simulink model "main_RI_LIEKF_GNSSOutrage"  (R2023a)
settings: Solver=FixedStepAuto  StartTime=0.0  StopTime=220  FixedStep=0.01  RelTol=1e-3
InitFcn:
  | initNavigation0612_AOA;
values from neighbouring files (symbols this model uses):
  CF_enable = 0    [initNavigation.m]
  dt = 0.01    [initNavigation.m]
  dtDelay = -0.03    [initNavigation.m]
  g0 = 9.795    [initNavigation.m]
  gam0_rad = 0/57.3    (= 0)    [initNavigation.m]
  GNSSoutragetime = 90    [initNavigation.m]
  H_sensor_type = 0    [initNavigation.m]
  KF_enable = 1    [initNavigation.m]
  P0 = diag([1*ones(3,1);0.01*ones(3,1);0.1*ones(3,1);0.001*ones(3,1);0.00001*ones(3,1)])    [initNavigation.m]
  P0_RIEKF = diag([1*ones(3,1);0.01*ones(3,1);0.1*ones(3,1);0.001*ones(3,1);0.00001*ones(3,1);      0.01*ones(3,1);[0;2;2]/57.3;[0.1;0.1;0.1]])^2    [initNavigation.m]
  pd0 = 0    [initNavigation.m]
  pe0 = 0    [initNavigation.m]
  phi0_rad = 0/57.3    (= 0)    [initNavigation.m]
  pn0 = 0    [initNavigation.m]
  psi = -178    [initNavigation.m]
  psi0_rad = 0/57.3    (= 0)    [initNavigation.m]
  state_dim = 24    [initNavigation.m]
  Time = 0:0.01:(size(traindata.AttackAngle,1) - 1)*0.01    [NNLiftCoefficientFit.m]
  vd0 = 0    [initNavigation.m]
  ve0 = 0    [initNavigation.m]
  vn0 = 0    [initNavigation.m]
undefined symbols (not defined in the file or in its folder): DiscIntNeverNeededParam, Discrete, INS_CONST, INS_EXPORT, INS_PARAM, magnitude, p, param, pInitialization, sys
libraries: simulink_extras x94, simulink x82, dspstat3 x70, sharedtransform x60, ctrlSharedLib x36, sharedTrackingLibrary x22, matrix_library x15, FMT_Model_Lib x13, deeplib x8, dspsolvers x4, vrlib x4, aerolibconvert2 x1
(part 15 of 28)

== system main_RI_LIEKF_GNSSOutrage/State estimation/distribute CF/distribute CF/AHRS1 ==
  RF_Data : Inport
  Sensor_Data : Inport  Port=2
  Bus_Constructor : Subsystem  TreatAsAtomicUnit=on
  Correct : Subsystem  TreatAsAtomicUnit=on
  Delay : Delay  DelayLength=1
  Update : Subsystem  TreatAsAtomicUnit=on
  Rotation_Data : Outport
  wires:
  Correct/1(att_B_correction) -> Update/1(att_B_correction)
  Bus_Constructor/1(Rotation_Data) -> Delay/1, Rotation_Data/1
  Correct/2(bias_g_B_correction) -> Update/2(bias_g_correction)
  Sensor_Data/1 -> Bus_Constructor/5(Sensor_Data), Update/4(Sensor_Data), Correct/2(Sensor_Data)
  Update/1(att_quat) -> Bus_Constructor/2(att_quat)
  Update/2(DCM_OB) -> Bus_Constructor/3(DCM_OB)
  Update/3(bias_g) -> Bus_Constructor/4(bias_g)
  RF_Data/1 -> Correct/3(RF_Data), Bus_Constructor/1(RF_Data), Update/3(RF_Data)
  Delay/1 -> Correct/1(Rotation_Data)

== system main_RI_LIEKF_GNSSOutrage/State estimation/distribute CF/distribute CF/Bus_Constructor ==
  RF_Data : Inport
  att_quat : Inport  Port=2
  DCM_OB : Inport  Port=3
  bias_g : Inport  Port=4
  gyro_B_correction : Inport  Port=5
  Sensor_Data : Inport  Port=6
  Bus Creator : BusCreator  Inputs=12
  Bus Selector : BusSelector  OutputSignals=IMU_Data.gyro_B_rad/s_LPF,IMU_Data.accl_B_m/s2_LPF
  Bus Selector1 : BusSelector  OutputSignals=att_reset
  Constant : Constant
  Euler_Angle : Subsystem
  Math Function : Math  Operator=transpose  SignedPower=on
  Signal Conversion{,1..4} (5 alike) : SignalConversion  OverrideOpt=off
  Subsystem1 : Subsystem
  Terminator2 : Terminator
  Rotation_Data : Outport
  wires:
  Bus Selector1/1 -> Signal Conversion4/1  "<att_reset>"
  Signal Conversion/1 -> Bus Creator/11  "acc_B_mPs2"
  Euler_Angle/1(phi_rad) -> Bus Creator/2  "phi_rad"
  Euler_Angle/2(theta_rad) -> Bus Creator/3  "theta_rad"
  Euler_Angle/3(psi_rad) -> Subsystem1/1(psi), Bus Creator/4  "psi_rad"
  Sensor_Data/1 -> Bus Selector/1
  Bus Creator/1 -> Rotation_Data/1
  bias_g/1 -> Signal Conversion3/1
  Math Function/1 -> Bus Creator/7  "M_BO"
  DCM_OB/1 -> Math Function/1, Bus Creator/8  "M_OB"
  att_quat/1 -> Euler_Angle/1(att_quat), Bus Creator/6  "att_quat"
  Subsystem1/1(DCMz) -> Bus Creator/5  "M_CO"
  Signal Conversion1/1 -> Bus Creator/12  "standstill"
  Bus Selector/2 -> Signal Conversion/1  "<accl_B_m/s2_LPF>"
  Signal Conversion2/1 -> Bus Creator/10  "gyr_B_radPs"
  Signal Conversion3/1 -> Bus Creator/9  "bias_g"
  RF_Data/1 -> Bus Selector1/1  "att_reset"
  gyro_B_correction/1 -> Signal Conversion2/1
  Signal Conversion4/1 -> Bus Creator/1  "att_reset"
  Constant/1 -> Signal Conversion1/1
  Bus Selector/1 -> Terminator2/1  "<gyro_B_rad/s_LPF>"

== system main_RI_LIEKF_GNSSOutrage/State estimation/distribute CF/distribute CF/Correct ==
  Sensor_Data : Inport
  Rotation_Data : Inport  Port=2
  Attitude_Correction : Subsystem
  Subsystem2 : Subsystem
  att_B_correction : Outport
  bias_g_B_correction : Outport  Port=2
  wires:
  Attitude_Correction/1(att_B_correction) -> att_B_correction/1, Subsystem2/2(att_B_correction)
  Sensor_Data/1 -> Subsystem2/1(Sensor_Data), Attitude_Correction/1(Sensor_Data)
  Subsystem2/1(bias_g_B_correction) -> bias_g_B_correction/1
  Rotation_Data/1 -> Attitude_Correction/2(Rotation_Data)

== system main_RI_LIEKF_GNSSOutrage/State estimation/distribute CF/distribute CF/Translation_estimate ==
  RotationData : Inport
  Sensor_data : Inport  Port=2
  Add : Sum  Inputs=++-
  Bus Creator2 : BusCreator  Inputs=6
  Bus Selector : BusSelector  OutputSignals=TOF_Data.H_TOF_TD,GPS_Data.pos_D_gps,QGC_sensor_reinit,GPS_Data.fixtype_gps
  Bus Selector1 : BusSelector  OutputSignals=M_OB
  Compare To Constant : simulink/Logic and Bit Operations/Compare To Constant  relop=>=  const=1  OutDataTypeStr=boolean
  Constant2 : Constant  Value=g0  OutDataTypeStr=single
  Demux : Demux  Outputs=2
  Demux1 : Demux  Outputs=2
  Demux2 : Demux  Outputs=3
  Detect Increase : simulink/Logic and Bit Operations/Detect Increase  vinit=0.0  OutDataTypeStr=boolean
  Gain : Gain  Gain=-1
  KalmanFilter_altitude : ctrlSharedLib/Kalman Filter  TimeDomain=Discrete-Time  UseCurrentEstimator=on  ModelSource=Individual A, B, C, D matrices  ModelSourceVariable=sys  A=[1 0.01 0; 0 1 -0.01;0 0 1-1/50;]  B=[0;0.01;0]  C=[1 0 0]  D=[0]  NumberOfStates=2  NumberOfInputs=2  NumberOfOutputs=2  InitialEstimateSource=Dialog  X0=[0 0 0]  P0=10  UseK=off  UseGH=on  NumberOfProcessNoiseInputs=2  G=diag([0;1;1])  TimeInvariantG=on  H=0  TimeInvariantH=on  Q=diag([0;5e-3;5e-4])  TimeInvariantQ=on  R=10  TimeInvariantR=on  N=0  TimeInvariantN=on  AddInputPort=on  AddEnablePort=on  ExternalReset=Rising  OutputEstimatedY=off  OutputP=off  Ts=-1
  Memory : Memory
  Rxy_Horizontal_estimation : Subsystem
  Scope : Scope  NumInputPorts=2
  Sensor_data1 : InportShadow  Port=2
  V_Horizontal_estimation : Subsystem
  Zero-Order Hold{,1..3} (4 alike) : ZeroOrderHold  SampleTime=0.01
  translate to N : Subsystem
  TranslationData : Outport
  wires:
  RotationData/1 -> Bus Selector1/1, translate to N/1(RotationData)
  Bus Creator2/1 -> TranslationData/1
  Demux1/2 -> Bus Creator2/5  "pe_m"
  Demux1/1 -> Bus Creator2/4  "pn_m"
  Demux/2 -> Bus Creator2/2  "ve_m/s"
  Demux/1 -> Bus Creator2/1  "vn_m/s"
  translate to N/2(accel_Vertical_predict) -> [accel_Vertical_predict]
  V_Horizontal_estimation/3(GPS_v_enable) -> Rxy_Horizontal_estimation/2(Enable)
  V_Horizontal_estimation/2(V_n&e) -> Rxy_Horizontal_estimation/1(Vn)
  V_Horizontal_estimation/1(vxy_estimout) -> Demux/1  "v_ne_"
  translate to N/1(accel_Horizontal_predict) -> V_Horizontal_estimation/1(An)
  Rxy_Horizontal_estimation/1(R_n&e) -> Demux1/1
  Sensor_data/1 -> translate to N/2(Sensor_data), V_Horizontal_estimation/2(Sensor_data2), Rxy_Horizontal_estimation/3(Sensor_data2)
  Sensor_data1/1 -> Bus Selector/1
  KalmanFilter_altitude/1 -> Demux2/1
  Demux2/1 -> Gain/1
  Zero-Order Hold/1 -> KalmanFilter_altitude/1
  Zero-Order Hold1/1 -> KalmanFilter_altitude/2
  Demux2/2 -> Bus Creator2/3  "vd_m/s"
  Gain/1 -> Bus Creator2/6  "H_m"
  [accel_Vertical_predict] -> Scope/1, Add/1
  Add/1 -> Zero-Order Hold/1
  Demux2/3 -> Memory/1
  Memory/1 -> Add/3, Scope/2
  Constant2/1 -> Add/2
  Bus Selector/3 -> Detect Increase/1  "<QGC_sensor_reinit>"
  Detect Increase/1 -> Zero-Order Hold3/1
  Bus Selector/4 -> Zero-Order Hold2/1  "<fixtype_gps>"
  Compare To Constant/1 -> KalmanFilter_altitude/3
  Zero-Order Hold2/1 -> Compare To Constant/1
  Bus Selector/2 -> Zero-Order Hold1/1  "<pos_D_gps>"
  Zero-Order Hold3/1 -> KalmanFilter_altitude/4
  Bus Selector1/1 -> Rxy_Horizontal_estimation/4(Cbn)  "<M_OB>"

== system main_RI_LIEKF_GNSSOutrage/State estimation/distribute CF/distribute CF/Update ==
  note: 比例环节
  att_B_correction : Inport
  bias_g_correction : Inport  Port=2
  RF_Data : Inport  Port=3
  Sensor_Data : Inport  Port=4
  Attitude_Update : Subsystem
  Bus Selector : BusSelector  OutputSignals=IMU_Data.gyro_B_rad/s_LPF
  Bus Selector1 : BusSelector  OutputSignals=att_reset,quat_0
  Gain : Gain
  Gyro_Bias_Update : Subsystem
  Saturation : Saturate  UpperLimit=0.1  LowerLimit=-0.1
  Scope : Scope
  Scope1 : Scope
  Sum2 : Sum  Inputs=|++
  att_quat : Outport
  DCM_OB : Outport  Port=2
  bias_g : Outport  Port=3
  gyro_B_correction : Outport  Port=4
  wires:
  Sensor_Data/1 -> Bus Selector/1
  Sum2/1 -> Attitude_Update/3(att_B_correction)
  Bus Selector/1 -> Gyro_Bias_Update/2(gyr_B_radPs)  "<gyro_B_rad/s_LPF>"
  bias_g_correction/1 -> Gyro_Bias_Update/1(bias_g_correction)
  Attitude_Update/1(att_quat) -> att_quat/1
  Attitude_Update/2(DCM_OB) -> DCM_OB/1
  Gyro_Bias_Update/2(bias_g) -> Scope/1, bias_g/1
  RF_Data/1 -> Bus Selector1/1  "att_reset"
  Bus Selector1/1 -> Attitude_Update/1(att_reset)  "<att_reset>"
  Bus Selector1/2 -> Attitude_Update/2(quat_0)  "<quat_0>"
  Gyro_Bias_Update/1(gyr_B_correction) -> gyro_B_correction/1, Sum2/2
  att_B_correction/1 -> Gain/1
  Gain/1 -> Saturation/1, Scope1/1
  Saturation/1 -> Sum2/1

== system main_RI_LIEKF_GNSSOutrage/State estimation/distribute CF/distribute CF/初始化 ==
  Sensor_Data : Inport
  Attitude_Reset : Subsystem
  Bus Creator : BusCreator  Inputs=2
  Scope : Scope
  Scope1 : Scope
  Subsystem : Subsystem
  RF_data : Outport
  wires:
  Attitude_Reset/1(att_reset) -> Subsystem/Enable, Bus Creator/1, Scope/1  "att_reset"
  Bus Creator/1 -> RF_data/1
  Subsystem/1(quat_0) -> Scope1/1, Bus Creator/2  "quat_0"
  Sensor_Data/1 -> Subsystem/1(sensor_data), Attitude_Reset/1(Sensor_Data)

== system main_RI_LIEKF_GNSSOutrage/Sensor_Data_Process/Magn_Data_Process1/Mag_Data_Process/Mag_Quality_Estimate/Mag_Quality ==
  nominal_inc_deg : Inport
  mag_normalized_O : Inport  Port=2
  Inclination_Quality_Estimate : Subsystem
  Intensity_Quality_Estimate : Subsystem
  MinMax : MinMax  Inputs=2
  低通滤波 : Subsystem  mask{fc=5, zeta=0.707}
      mask prompts: fc "Cut-off frequence"; zeta "Damping factor"
      mask DialogControl ParameterGroupVar Prompt: 参数
  mag_quality : Outport  PortDimensions=1  VectorParamsAs1DForOutWhenUnconnected=off
  wires:
  Intensity_Quality_Estimate/1(intensity_quality) -> MinMax/2  "mag_int_quality"
  nominal_inc_deg/1 -> Inclination_Quality_Estimate/1(nominal_inc_deg)
  Inclination_Quality_Estimate/1(inclination_quality) -> MinMax/1  "mag_inc_quality"
  mag_normalized_O/1 -> Inclination_Quality_Estimate/2(mag_normalized_O), Intensity_Quality_Estimate/1(mag_normalized_O)
  MinMax/1 -> 低通滤波/1(u)
  低通滤波/1(y) -> mag_quality/1

== system main_RI_LIEKF_GNSSOutrage/Sensor_Data_Process/Magn_Data_Process1/Mag_Data_Process/WMM_Compensation/Normlize ==
  In1 : Inport
  Constant : Constant  OutDataTypeStr=Inherit: Inherit via back propagation
  Data Type Duplicate : DataTypeDuplicate
  Demux : Demux  Outputs=[-1 1]
  Divide : Product  Inputs=*/
  Ground : Ground
  Math Function : Math  Operator=square  SignedPower=on  OutDataTypeStr=Inherit: Inherit via internal rule
  Math Function1 : Math  Operator=sqrt  SignedPower=on
  Mux : Mux  Inputs=2
  Mux1 : Mux  Inputs=2
  Product : Product  RndMeth=Zero  OutDataTypeStr=Inherit: Same as first input
  Sum of Elements : Sum  Inputs=+
  Switch : Switch  Criteria=u2 > Threshold  SaturateOnIntegerOverflow=off  InputSameDT=off
  Out1 : Outport  PortDimensions=3
  wires:
  Mux/1 -> Switch/1
  Ground/1 -> Product/2
  In1/1 -> Mux/1, Math Function/1, Product/1, Data Type Duplicate/2
  Sum of Elements/1 -> Math Function1/1
  Product/1 -> Mux1/1
  Math Function1/1 -> Switch/2, Mux/2
  Demux/2 -> Divide/2
  Switch/1 -> Demux/1
  Mux1/1 -> Switch/3
  Math Function/1 -> Sum of Elements/1
  Constant/1 -> Mux1/2, Data Type Duplicate/1
  Demux/1 -> Divide/1
  Divide/1 -> Out1/1

== system main_RI_LIEKF_GNSSOutrage/Sensor_Data_Process/Magn_Data_Process1/Mag_Data_Process/WMM_Compensation/psi2DCMz ==
  In1 : Inport
  Constant : Constant  OutDataTypeStr=Inherit: Inherit via back propagation
  Constant{1..4} (4 alike) : Constant  Value=0  OutDataTypeStr=Inherit: Inherit via back propagation
  Gain1 : Gain  Gain=-1
  Trigonometric Function : Trigonometry
  Trigonometric Function1 : Trigonometry  Operator=cos
  Trigonometric Function2 : Trigonometry
  Trigonometric Function3 : Trigonometry  Operator=cos
  Vector Concatenate : Concatenate  NumInputs=3  Mode=Multidimensional array  ConcatenateDimension=2
  Vector Concatenate1 : Concatenate  NumInputs=3  Mode=Multidimensional array
  Vector Concatenate2 : Concatenate  NumInputs=3  Mode=Multidimensional array
  Vector Concatenate3 : Concatenate  NumInputs=3  Mode=Multidimensional array
  Out1 : Outport
  wires:
  Constant1/1 -> Vector Concatenate3/2
  Constant/1 -> Vector Concatenate3/3
  Vector Concatenate/1 -> Out1/1
  Trigonometric Function2/1 -> Gain1/1
  Constant2/1 -> Vector Concatenate3/1
  In1/1 -> Trigonometric Function3/1, Trigonometric Function2/1, Trigonometric Function/1, Trigonometric Function1/1
  Trigonometric Function/1 -> Vector Concatenate1/2
  Vector Concatenate2/1 -> Vector Concatenate/2
  Vector Concatenate1/1 -> Vector Concatenate/1
  Vector Concatenate3/1 -> Vector Concatenate/3
  Gain1/1 -> Vector Concatenate2/1
  Constant3/1 -> Vector Concatenate1/3
  Trigonometric Function1/1 -> Vector Concatenate1/1
  Constant4/1 -> Vector Concatenate2/3
  Trigonometric Function3/1 -> Vector Concatenate2/2

== system main_RI_LIEKF_GNSSOutrage/Sensor_Data_Process/Magn_Data_Process1/Mag_Data_Process/WMM_Compensation/safe_divide ==
  u1 : Inport
  u2 : Inport  Port=2
  Constant1 : Constant  VectorParams1D=off  OutDataTypeStr=single
  Divide1 : Product  Inputs=*/
  MinMax : MinMax  Function=max  Inputs=2
  y : Outport  VectorParamsAs1DForOutWhenUnconnected=off
  wires:
  MinMax/1 -> Divide1/2
  Constant1/1 -> MinMax/1
  Divide1/1 -> y/1
  u2/1 -> MinMax/2
  u1/1 -> Divide1/1

== system main_RI_LIEKF_GNSSOutrage/State estimation/0609bk/Error State Kalman Filter/Extended Kalman Filter1/Correct1 ==
  yMeas : Inport  SampleTime=SampleTime
  R : Inport  Port=2  SampleTime=SampleTime
  uMeas : Inport  Port=3  SampleTime=SampleTime
  uBlockOrdering : Inport  Port=4  SampleTime=SampleTime
  Enable : EnablePort
  Correct : MATLAB Function  TreatAsAtomicUnit=on
  Data Store ReadP : DataStoreRead  DataStoreName=P  IndexOptions=Index vector (dialog)  Indices=1  OutputSizes=1
  Data Store ReadX : DataStoreRead  DataStoreName=x  IndexOptions=Index vector (dialog)  Indices=1  OutputSizes=1
  Data Store WriteP : DataStoreWrite  DataStoreName=P  IndexOptions=Index vector (dialog)  Indices=1  OutputSizes=1
  Data Store WriteX : DataStoreWrite  DataStoreName=x  IndexOptions=Index vector (dialog)  Indices=1  OutputSizes=1
  IGG_check : Subsystem  Commented=on
  R1 : InportShadow  Port=2  SampleTime=SampleTime
  RegisterSimulinkFcn : S-Function  FunctionName=ekfukfRegisterSimulinkFcn  Parameters=int32(3), 1, pM.HasAdditiveNoise, SampleTime, DataType, SLFcnsToRegister  SFunctionDeploymentMode=off  EnableBusSupport=off
  Scope1 : Scope
  yMeas1 : InportShadow  SampleTime=SampleTime
  yBlockOrdering : Outport  VectorParamsAs1DForOutWhenUnconnected=off
  wires:
  uMeas/1 -> Correct/5(uMeas)
  uBlockOrdering/1 -> Correct/6("blockOrdering ")
  Correct/3(blockOrdering) -> yBlockOrdering/1
  Correct/1(xNew) -> Data Store WriteX/1
  R/1 -> RegisterSimulinkFcn/3, Correct/4(R)
  yMeas/1 -> RegisterSimulinkFcn/2, Correct/3(yMeas)
  Correct/2(P) -> Data Store WriteP/1
  Data Store ReadP/1 -> IGG_check/1(Pk/k_1), Correct/2("P ")
  Data Store ReadX/1 -> IGG_check/3(X), Correct/1(x), RegisterSimulinkFcn/1
  yMeas1/1 -> IGG_check/2(yMeas)
  R1/1 -> IGG_check/4(R)
  IGG_check/2(w) -> Scope1/1

== system main_RI_LIEKF_GNSSOutrage/State estimation/0609bk/Error State Kalman Filter/Extended Kalman Filter1/Output ==
  uBlockOrdering : Inport
  Data Store Read : DataStoreRead  DataStoreName=x  IndexOptions=Index vector (dialog)  Indices=1  OutputSizes=1
  Data Store Read1 : DataStoreRead  DataStoreName=P  IndexOptions=Index vector (dialog)  Indices=1  OutputSizes=1
  MATLAB Function : MATLAB Function  TreatAsAtomicUnit=on
  x : Outport  VectorParamsAs1DForOutWhenUnconnected=off
  P : Outport  Port=2  VectorParamsAs1DForOutWhenUnconnected=off
  yBlockOrdering : Outport  Port=3  VectorParamsAs1DForOutWhenUnconnected=off
  wires:
  MATLAB Function/1(P) -> P/1
  uBlockOrdering/1 -> yBlockOrdering/1
  Data Store Read1/1 -> MATLAB Function/1(S)
  Data Store Read/1 -> x/1

== system main_RI_LIEKF_GNSSOutrage/State estimation/0609bk/Error State Kalman Filter/Extended Kalman Filter1/Predict ==
  Q : Inport  SampleTime=SampleTime
  uState : Inport  Port=2  SampleTime=SampleTime
  uBlockOrdering : Inport  Port=3  SampleTime=SampleTime
  Data Store Read1 : DataStoreRead  Commented=on  DataStoreName=feedback_flag_18dim  IndexOptions=Index vector (dialog)  Indices=1  OutputSizes=1
  Data Store Write : DataStoreWrite  DataStoreName=P  IndexOptions=Index vector (dialog)  Indices=1  OutputSizes=1
  Data Store Write1 : DataStoreWrite  DataStoreName=x  IndexOptions=Index vector (dialog)  Indices=1  OutputSizes=1
  Data Store WriteX : DataStoreWrite  DataStoreName=x  IndexOptions=Index vector (dialog)  Indices=1  OutputSizes=1
  Data Store ReadP : DataStoreRead  DataStoreName=P  IndexOptions=Index vector (dialog)  Indices=1  OutputSizes=1
  Data Store ReadX : DataStoreRead  DataStoreName=x  IndexOptions=Index vector (dialog)  Indices=1  OutputSizes=1
  If : If  Commented=on  IfExpression=u1 == 1  ShowElse=off
  If Action Subsystem : Subsystem  Commented=on  TreatAsAtomicUnit=on
  Predict : MATLAB Function  TreatAsAtomicUnit=on
  RegisterSimulinkFcn : S-Function  FunctionName=ekfukfRegisterSimulinkFcn  Parameters=int32(2), 0, pS.HasAdditiveNoise, SampleTime, DataType, SLFcnsToRegister  SFunctionDeploymentMode=off  EnableBusSupport=off
  Zero : Constant  Value=zeros(15,1)  OutDataTypeStr=Inherit: Inherit via back propagation
  wires:
  Zero/1 -> Data Store Write1/1
  If/1 -> If Action Subsystem/Action
  Data Store Read1/1 -> If/1
  uState/1 -> Predict/4(uState)
  uBlockOrdering/1 -> Predict/5(unused)
  Data Store ReadX/1 -> RegisterSimulinkFcn/1, Predict/1(x)
  Predict/1(xNew) -> Data Store WriteX/1
  Q/1 -> RegisterSimulinkFcn/2, Predict/3(Q)
  Predict/2(P) -> Data Store Write/1
  Data Store ReadP/1 -> Predict/2("P ")

== system main_RI_LIEKF_GNSSOutrage/State estimation/0609bk/Error State Kalman Filter/Simulink Function - State Transition/Cal Phi ==
  Rbn : Inport
  vn : Inport  Port=2
  pn : Inport  Port=3
  Constant : Constant  Value=dt
  MATLAB Function1 : MATLAB Function  TreatAsAtomicUnit=on
  Reshape : Reshape  OutputDimensionality=Column vector (2-D)
  Reshape1 : Reshape  OutputDimensionality=Column vector (2-D)
  Phi : Outport
  wires:
  Reshape1/1 -> MATLAB Function1/2(pn)
  Reshape/1 -> MATLAB Function1/1(vn)
  pn/1 -> Reshape1/1
  vn/1 -> Reshape/1
  Rbn/1 -> MATLAB Function1/3(Rbn)
  MATLAB Function1/1(Phi) -> Phi/1
  Constant/1 -> MATLAB Function1/4(dt)

== system main_RI_LIEKF_GNSSOutrage/State estimation/0609bk/INS propogation/Init_PVQ/Horizontal_attitude ==
  note: fai
  note: gamma
  accl_mean_B_m/s_LPF : Inport  PortDimensions=3
  Magn_mean_B_guess_LPF : Inport  Port=2
  Enable : EnablePort
  Add : Sum  Inputs=+-
  Asin : Trigonometry  Operator=asin
  Atan2 : Trigonometry  Operator=atan2
  Data Type Conversion : DataTypeConversion  SaturateOnIntegerOverflow=off  RndMeth=Floor
  Deal with zero : Subsystem
  Degrees to Radians : simulink_extras/Transformations/Degrees to Radians
  Degrees to Radians1 : simulink_extras/Transformations/Degrees to Radians
  Demux : Demux  Outputs=3
  Divide : Product  Inputs=*/  OutDataTypeStr=single
  Gain1 : Gain  Gain=-1
  Gain2 : Gain  Gain=-1
  Magnetic declination : Constant  Value=param.fusion.magDeclDeg  OutDataTypeStr=single
  Magnetic declination1 : Constant  Value=param.control.MagnheadingCorrection  OutDataTypeStr=uint8
  Math Function : Math  Operator=magnitude^2  SignedPower=on
  Mux : Mux  Inputs=3
  Mux1 : Mux  Inputs=3
  Mux3 : Mux  Inputs=3
  Product : Product  Multiplication=Matrix(*)
  Quaternions to Direction Cosine Matrix : sharedtransform/Quaternions to  Direction Cosine Matrix  aMode=aMode
  Rotation Angles to Quaternions : sharedtransform/Rotation Angles to Quaternions  rotationOrder=ZYX  aMode=aMode
  Rotation Angles to Quaternions1 : sharedtransform/Rotation Angles to Quaternions  rotationOrder=ZYX  aMode=aMode
  Scope : Scope
  Scope1 : Scope
  Selector : Selector  InputPortWidth=3  IndexOptions=Index vector (dialog)  Indices=[2]  OutputSizes=1
  Selector1 : Selector  InputPortWidth=3  IndexOptions=Index vector (dialog)  Indices=[1]  OutputSizes=1
  Sqrt : Sqrt
  Sum of Elements : Sum  Inputs=+
  Switch : Switch  Threshold=0.5  SaturateOnIntegerOverflow=off  InputSameDT=off
  Terminator : Terminator
  Transpose : Math  Operator=transpose  SignedPower=on
  Trigonometric Function1 : Trigonometry  Operator=atan2
  psi_zero : Constant  Value=psi  OutDataTypeStr=single
  quat_0 : Outport  PortDimensions=4
  wires:
  Rotation Angles to Quaternions1/1 -> Switch/1
  accl_mean_B_m/s_LPF/1 -> Demux/1
  Sqrt/1 -> Deal with zero/1(In1)
  Deal with zero/1(Out1) -> Divide/2
  Trigonometric Function1/1 -> Gain2/1
  Demux/1 -> Divide/1, Mux/2
  Demux/2 -> Mux/1, Trigonometric Function1/1
  Demux/3 -> Gain1/1
  Sum of Elements/1 -> Sqrt/1
  Divide/1 -> Asin/1
  Mux/1 -> Math Function/1
  Math Function/1 -> Sum of Elements/1
  Mux1/1 -> Rotation Angles to Quaternions/1
  psi_zero/1 -> Degrees to Radians1/1
  Asin/1 -> Mux3/2, Mux1/2
  Gain2/1 -> Mux3/3, Mux1/3
  Rotation Angles to Quaternions/1 -> Switch/3, Quaternions to Direction Cosine Matrix/1  "q0_no_yaw"
  Quaternions to Direction Cosine Matrix/1 -> Transpose/1
  Magn_mean_B_guess_LPF/1 -> Product/2
  Product/1 -> Selector/1, Selector1/1  "magNED"
  Selector1/1 -> Atan2/2  "magN"
  Selector/1 -> Atan2/1  "magE"
  Atan2/1 -> Add/2
  Magnetic declination/1 -> Degrees to Radians/1
  Add/1 -> Mux3/1  "psi_calbymag"
  Mux3/1 -> Rotation Angles to Quaternions1/1
  Transpose/1 -> Product/1
  Gain1/1 -> Trigonometric Function1/2, Mux/3
  Degrees to Radians1/1 -> Mux1/1
  Degrees to Radians/1 -> Terminator/1
  Magnetic declination1/1 -> Data Type Conversion/1, Switch/2
  Switch/1 -> Scope1/1, quat_0/1
  Data Type Conversion/1 -> Scope/1

== system main_RI_LIEKF_GNSSOutrage/State estimation/0609bk/INS propogation/Init_PVQ/Subsystem ==
  data : Inport
  Buffer : Buffer  N=50  V=49  OutputFrames=off
  Buffer1 : Buffer  N=50  V=49  OutputFrames=off
  Buffer2 : Buffer  N=50  V=49  ic=-g0  OutputFrames=off
  Demux : Demux  Outputs=3
  Mean4 : dspstat3/Mean  run=off  reset_popup=None  directionMode=Entire input  dimension=3  roiEnable=off  roiType=Rectangles  roiPortion=Entire ROI  roiOutput=Individual statistics for each ROI  roiFlag=off  roundingMode=Floor  overflowMode=off  outputDataTypeStr=Inherit: Same as accumulator  outputMin=[]  outputMax=[]  outputLastDataTypeStr=Inherit: Same as accumulator
  Mean5 : dspstat3/Mean  run=off  reset_popup=None  directionMode=Entire input  dimension=3  roiEnable=off  roiType=Rectangles  roiPortion=Entire ROI  roiOutput=Individual statistics for each ROI  roiFlag=off  roundingMode=Floor  overflowMode=off  outputDataTypeStr=Inherit: Same as accumulator  outputMin=[]  outputMax=[]  outputLastDataTypeStr=Inherit: Same as accumulator
  Mean6 : dspstat3/Mean  run=off  reset_popup=None  directionMode=Entire input  dimension=3  roiEnable=off  roiType=Rectangles  roiPortion=Entire ROI  roiOutput=Individual statistics for each ROI  roiFlag=off  roundingMode=Floor  overflowMode=off  outputDataTypeStr=Inherit: Same as accumulator  outputMin=[]  outputMax=[]  outputLastDataTypeStr=Inherit: Same as accumulator
  Scope : Scope  NumInputPorts=2
  Vector Concatenate : Concatenate  NumInputs=3
  mean_data : Outport
  wires:
  Mean6/1 -> Vector Concatenate/3
  Demux/2 -> Buffer1/1
  Buffer/1 -> Mean4/1  "fbx_buff"
  Mean5/1 -> Vector Concatenate/2
  Buffer2/1 -> Mean6/1  "fbz_buff"
  Demux/1 -> Buffer/1
  Buffer1/1 -> Mean5/1  "fby_buff"
  Demux/3 -> Buffer2/1
  Mean4/1 -> Vector Concatenate/1
  Vector Concatenate/1 -> Scope/2, mean_data/1
  data/1 -> Scope/1, Demux/1

== system main_RI_LIEKF_GNSSOutrage/State estimation/0609bk/INS propogation/Init_PVQ/Subsystem1 ==
  data : Inport
  Buffer : Buffer  N=50  V=49  OutputFrames=off
  Buffer1 : Buffer  N=50  V=49  OutputFrames=off
  Buffer2 : Buffer  N=50  V=49  OutputFrames=off
  Demux : Demux  Outputs=3
  Mean4 : dspstat3/Mean  run=off  reset_popup=None  directionMode=Entire input  dimension=3  roiEnable=off  roiType=Rectangles  roiPortion=Entire ROI  roiOutput=Individual statistics for each ROI  roiFlag=off  roundingMode=Floor  overflowMode=off  outputDataTypeStr=Inherit: Same as accumulator  outputMin=[]  outputMax=[]  outputLastDataTypeStr=Inherit: Same as accumulator
  Mean5 : dspstat3/Mean  run=off  reset_popup=None  directionMode=Entire input  dimension=3  roiEnable=off  roiType=Rectangles  roiPortion=Entire ROI  roiOutput=Individual statistics for each ROI  roiFlag=off  roundingMode=Floor  overflowMode=off  outputDataTypeStr=Inherit: Same as accumulator  outputMin=[]  outputMax=[]  outputLastDataTypeStr=Inherit: Same as accumulator
  Mean6 : dspstat3/Mean  run=off  reset_popup=None  directionMode=Entire input  dimension=3  roiEnable=off  roiType=Rectangles  roiPortion=Entire ROI  roiOutput=Individual statistics for each ROI  roiFlag=off  roundingMode=Floor  overflowMode=off  outputDataTypeStr=Inherit: Same as accumulator  outputMin=[]  outputMax=[]  outputLastDataTypeStr=Inherit: Same as accumulator
  Vector Concatenate : Concatenate  NumInputs=3
  mean_data : Outport
  wires:
  data/1 -> Demux/1
  Vector Concatenate/1 -> mean_data/1
  Mean4/1 -> Vector Concatenate/1
  Demux/3 -> Buffer2/1
  Buffer1/1 -> Mean5/1  "fby_buff"
  Demux/1 -> Buffer/1
  Buffer2/1 -> Mean6/1  "fbz_buff"
  Mean5/1 -> Vector Concatenate/2
  Buffer/1 -> Mean4/1  "fbx_buff"
  Demux/2 -> Buffer1/1
  Mean6/1 -> Vector Concatenate/3

== system main_RI_LIEKF_GNSSOutrage/State estimation/0609bk/INS propogation/vel_pos_update/Kinematic Equation ==
  Cbn : Inport
  Ab : Inport  Port=2
  Add : Sum  Inputs=+-
  Constant : Constant  Value=[0 0 -g0]  OutDataTypeStr=single
  Product : Product  Multiplication=Matrix(*)  RndMeth=Zero
  Scope : Scope
  Scope1 : Scope  NumInputPorts=2
  An : Outport
  wires:
  Cbn/1 -> Product/1
  Add/1 -> An/1, Scope1/2
  Ab/1 -> Product/2, Scope1/1
  Product/1 -> Scope/1, Add/1
  Constant/1 -> Add/2

== system main_RI_LIEKF_GNSSOutrage/State estimation/0609bk/INS propogation/vel_pos_update/pos update ==
  vel_k : Inport
  pn : Inport  Port=2
  QGC_init : Inport  Port=3
  p0 : Inport  Port=4
  Add1 : Sum
  Delay1 : Delay  DelayLength=1  InitialConditionSource=Input port  ExternalReset=Rising
      settings: InputPortMap=u0,r5,p4
  Gain1 : Gain  Gain=dt
  Reshape1 : Reshape  OutputDimensionality=Column vector (2-D)
  p_k : Outport
  wires:
  p0/1 -> Reshape1/1
  QGC_init/1 -> Delay1/2
  Reshape1/1 -> Delay1/3
  Delay1/1 -> Add1/2
  Gain1/1 -> Add1/1
  vel_k/1 -> Gain1/1
  Add1/1 -> p_k/1
  pn/1 -> Delay1/1

== system main_RI_LIEKF_GNSSOutrage/State estimation/0609bk/INS propogation/vel_pos_update/vel update ==
  QGC_init : Inport
  An : Inport  Port=2
  vn : Inport  Port=3
  v0 : Inport  Port=4
  Add : Sum
  Delay : Delay  DelayLength=1  InitialConditionSource=Input port  ExternalReset=Rising
      settings: InputPortMap=u0,r5,p4
  Gain : Gain  Gain=dt
  Reshape : Reshape  OutputDimensionality=Column vector (2-D)
  vel_k : Outport
  wires:
  QGC_init/1 -> Delay/2
  Reshape/1 -> Delay/3
  An/1 -> Gain/1
  v0/1 -> Reshape/1
  Gain/1 -> Add/1
  Delay/1 -> Add/2
  Add/1 -> vel_k/1
  vn/1 -> Delay/1

== system main_RI_LIEKF_GNSSOutrage/State estimation/15dim KF1/Error State Kalman Filter/GNSS//INS Kalman Filter1/CalculatePL ==
  A[k] : Inport  SampleTime=pInitialization.Ts
  C[k] : Inport  Port=2  SampleTime=pInitialization.Ts
  Qbar[k] : Inport  Port=3  SampleTime=pInitialization.Ts
  Rbar[k] : Inport  Port=4  SampleTime=pInitialization.Ts
  Nbar[k] : Inport  Port=5  SampleTime=pInitialization.Ts
  Enable[k] : Inport  Port=6  SampleTime=pInitialization.Ts
  P[k] : Inport  Port=7  SampleTime=pInitialization.Ts
  Discrete-Time KF - Calculate PLMZ : MATLAB Function  TreatAsAtomicUnit=on
  M[k] : Outport  SampleTime=pInitialization.Ts  VectorParamsAs1DForOutWhenUnconnected=off
  L[k] : Outport  Port=2  SampleTime=pInitialization.Ts  VectorParamsAs1DForOutWhenUnconnected=off
  Z[k] : Outport  Port=3  SampleTime=pInitialization.Ts  VectorParamsAs1DForOutWhenUnconnected=off
  P[k+1] : Outport  Port=4  SampleTime=pInitialization.Ts  VectorParamsAs1DForOutWhenUnconnected=off
  wires:
  A[k]/1 -> Discrete-Time KF - Calculate PLMZ/1(A)
  C[k]/1 -> Discrete-Time KF - Calculate PLMZ/2(C)
  Qbar[k]/1 -> Discrete-Time KF - Calculate PLMZ/3(Q)
  P[k]/1 -> Discrete-Time KF - Calculate PLMZ/6(P)
  Rbar[k]/1 -> Discrete-Time KF - Calculate PLMZ/4(R)
  Nbar[k]/1 -> Discrete-Time KF - Calculate PLMZ/5(N)
  Discrete-Time KF - Calculate PLMZ/1(L) -> L[k]/1
  Discrete-Time KF - Calculate PLMZ/4(PNew) -> P[k+1]/1
  Enable[k]/1 -> Discrete-Time KF - Calculate PLMZ/7(isEnabled)
  Discrete-Time KF - Calculate PLMZ/2(M) -> M[k]/1
  Discrete-Time KF - Calculate PLMZ/3(Z) -> Z[k]/1

== system main_RI_LIEKF_GNSSOutrage/State estimation/15dim KF1/Error State Kalman Filter/GNSS//INS Kalman Filter1/CovarianceOutputConfigurator ==
  Z : Inport
  P : Inport  Port=2
  TerminatorP : Terminator
  TerminatorZ : Terminator
  decideOutput : Subsystem  mask(outputZorP){}
  Covariance : Outport  VectorParamsAs1DForOutWhenUnconnected=off
  wires:
  decideOutput/1(P) -> Covariance/1
  P/1 -> TerminatorP/1, decideOutput/1(Z)
  Z/1 -> TerminatorZ/1

== system main_RI_LIEKF_GNSSOutrage/State estimation/15dim KF1/Error State Kalman Filter/GNSS//INS Kalman Filter1/If Action Subsystem1 ==
  x[k+1|k] : Inport
  Action Port : ActionPort
  Constant : Constant  Value=0
  Data Store Write : DataStoreWrite  DataStoreName=feedback_flag  IndexOptions=Index vector (dialog)  Indices=1  OutputSizes=1
  Gain : Gain  Gain=0
  Out1 : Outport
  wires:
  Constant/1 -> Data Store Write/1
  Gain/1 -> Out1/1
  x[k+1|k]/1 -> Gain/1

== system main_RI_LIEKF_GNSSOutrage/State estimation/15dim KF1/Error State Kalman Filter/GNSS//INS Kalman Filter1/If Action Subsystem2 ==
  x[k+1|k] : Inport
  Action Port : ActionPort
  Out1 : Outport
  wires:
  x[k+1|k]/1 -> Out1/1

== system main_RI_LIEKF_GNSSOutrage/State estimation/15dim KF1/Error State Kalman Filter/GNSS//INS Kalman Filter1/If Action Subsystem3 ==
  Action Port : ActionPort
  Constant : Constant  Value=0
  Data Store Write : DataStoreWrite  DataStoreName=feedback_flag  IndexOptions=Index vector (dialog)  Indices=1  OutputSizes=1
  wires:
  Constant/1 -> Data Store Write/1

== system main_RI_LIEKF_GNSSOutrage/State estimation/15dim KF1/Error State Kalman Filter/GNSS//INS Kalman Filter1/Observer ==
  note: A*xhat+B*u+L*(yMeas-yHat)
      | or
      | A*xhat+B*u
  u[k] : Inport  SampleTime=pInitialization.Ts
  y[k] : Inport  Port=2  SampleTime=pInitialization.Ts
  A[k] : Inport  Port=3  SampleTime=pInitialization.Ts
  B[k] : Inport  Port=4  SampleTime=pInitialization.Ts
  C[k] : Inport  Port=5  SampleTime=pInitialization.Ts
  D[k] : Inport  Port=6  SampleTime=pInitialization.Ts
  L[k] : Inport  Port=7  SampleTime=pInitialization.Ts
  Enable : Inport  Port=8  SampleTime=pInitialization.Ts
  xhat[k|k-1] : Inport  Port=9  SampleTime=pInitialization.Ts
  A[k]*xhat[k|k-1] : Product  Multiplication=Matrix(*)
  Add : Sum  Inputs=+++
  B[k]*u[k] : Product  Multiplication=Matrix(*)
  MeasurementUpdate : Subsystem  TreatAsAtomicUnit=on
  Reshape : Reshape
  x[k+1|k] : Outport  SampleTime=pInitialization.Ts  VectorParamsAs1DForOutWhenUnconnected=off
  wires:
  D[k]/1 -> MeasurementUpdate/5(D[k])
  Reshape/1 -> x[k+1|k]/1
  y[k]/1 -> MeasurementUpdate/2(y[k])
  C[k]/1 -> MeasurementUpdate/3(C[k])
  MeasurementUpdate/1(L*(y[k]-yhat[k|k-1])) -> Add/3
  A[k]/1 -> A[k]*xhat[k|k-1]/1
  xhat[k|k-1]/1 -> A[k]*xhat[k|k-1]/2, MeasurementUpdate/4(xhat[k|k-1])
  B[k]/1 -> B[k]*u[k]/1
  L[k]/1 -> MeasurementUpdate/1(L[k])
  A[k]*xhat[k|k-1]/1 -> Add/2
  u[k]/1 -> B[k]*u[k]/2, MeasurementUpdate/6(u[k])
  Add/1 -> Reshape/1
  B[k]*u[k]/1 -> Add/1
  Enable/1 -> MeasurementUpdate/Enable

== system main_RI_LIEKF_GNSSOutrage/State estimation/15dim KF1/INS propogation/Init_PVQ2/Horizontal_attitude ==
  note: gamma
  note: fai
  accl_mean_B_m/s_LPF : Inport  PortDimensions=3
  Magn_mean_B_guess_LPF : Inport  Port=2
  Enable : EnablePort
  Add : Sum  Inputs=+-
  Asin : Trigonometry  Operator=asin
  Atan2 : Trigonometry  Operator=atan2
  Data Type Conversion : DataTypeConversion  SaturateOnIntegerOverflow=off  RndMeth=Floor
  Deal with zero : Subsystem
  Degrees to Radians : simulink_extras/Transformations/Degrees to Radians
  Degrees to Radians1 : simulink_extras/Transformations/Degrees to Radians
  Demux : Demux  Outputs=3
  Divide : Product  Inputs=*/  OutDataTypeStr=single
  Gain1 : Gain  Gain=-1
  Gain2 : Gain  Gain=-1
  Hem2JPL : MATLAB Function  TreatAsAtomicUnit=on
  Hem2JPL1 : MATLAB Function  TreatAsAtomicUnit=on
  Magnetic declination : Constant  Value=param.fusion.magDeclDeg  OutDataTypeStr=single
  Magnetic declination1 : Constant  Value=param.control.MagnheadingCorrection  OutDataTypeStr=uint8
  Math Function : Math  Operator=magnitude^2  SignedPower=on
  Mux : Mux  Inputs=3
  Mux1 : Mux  Inputs=3
  Mux3 : Mux  Inputs=3
  Product : Product  Multiplication=Matrix(*)
  Quaternions to Direction Cosine Matrix : sharedtransform/Quaternions to  Direction Cosine Matrix  aMode=aMode
  Rotation Angles to Quaternions : sharedtransform/Rotation Angles to Quaternions  rotationOrder=ZYX  aMode=aMode
  Rotation Angles to Quaternions1 : sharedtransform/Rotation Angles to Quaternions  rotationOrder=ZYX  aMode=aMode
  Scope : Scope
  Scope1 : Scope
  Selector : Selector  InputPortWidth=3  IndexOptions=Index vector (dialog)  Indices=[2]  OutputSizes=1
  Selector1 : Selector  InputPortWidth=3  IndexOptions=Index vector (dialog)  Indices=[1]  OutputSizes=1
  Sqrt : Sqrt
  Sum of Elements : Sum  Inputs=+
  Switch : Switch  Threshold=0.5  SaturateOnIntegerOverflow=off  InputSameDT=off
  Terminator : Terminator
  Transpose : Math  Operator=transpose  SignedPower=on
  Trigonometric Function1 : Trigonometry  Operator=atan2
  psi_zero : Constant  Value=psi  OutDataTypeStr=single
  quat_0 : Outport  PortDimensions=4
  wires:
  Data Type Conversion/1 -> Scope/1
  Rotation Angles to Quaternions1/1 -> Hem2JPL1/1(q)
  Switch/1 -> quat_0/1, Scope1/1
  Magnetic declination1/1 -> Switch/2, Data Type Conversion/1
  Degrees to Radians/1 -> Terminator/1
  Degrees to Radians1/1 -> Mux1/1
  Gain1/1 -> Trigonometric Function1/2, Mux/3
  Transpose/1 -> Product/1
  Mux3/1 -> Rotation Angles to Quaternions1/1
  Add/1 -> Mux3/1  "psi_calbymag"
  Magnetic declination/1 -> Degrees to Radians/1
  Atan2/1 -> Add/2
  Selector/1 -> Atan2/1  "magE"
  Selector1/1 -> Atan2/2  "magN"
  Product/1 -> Selector1/1, Selector/1  "magNED"
  Magn_mean_B_guess_LPF/1 -> Product/2
  Quaternions to Direction Cosine Matrix/1 -> Transpose/1
  Rotation Angles to Quaternions/1 -> Hem2JPL/1(q)  "q0_no_yaw"
  Gain2/1 -> Mux1/3, Mux3/3
  Asin/1 -> Mux1/2, Mux3/2
  psi_zero/1 -> Degrees to Radians1/1
  Mux1/1 -> Rotation Angles to Quaternions/1
  Math Function/1 -> Sum of Elements/1
  Mux/1 -> Math Function/1
  Divide/1 -> Asin/1
  Sum of Elements/1 -> Sqrt/1
  Demux/3 -> Gain1/1
  Demux/2 -> Trigonometric Function1/1, Mux/1
  Demux/1 -> Mux/2, Divide/1
  Trigonometric Function1/1 -> Gain2/1
  Deal with zero/1(Out1) -> Divide/2
  Sqrt/1 -> Deal with zero/1(In1)
  accl_mean_B_m/s_LPF/1 -> Demux/1
  Hem2JPL/1(y) -> Quaternions to Direction Cosine Matrix/1, Switch/3
  Hem2JPL1/1(y) -> Switch/1

== system main_RI_LIEKF_GNSSOutrage/State estimation/15dim KF1/INS propogation/Init_PVQ2/Subsystem ==
  data : Inport
  Buffer : Buffer  N=50  V=49  OutputFrames=off
  Buffer1 : Buffer  N=50  V=49  OutputFrames=off
  Buffer2 : Buffer  N=50  V=49  ic=-g0  OutputFrames=off
  Demux : Demux  Outputs=3
  Mean4 : dspstat3/Mean  run=off  reset_popup=None  directionMode=Entire input  dimension=3  roiEnable=off  roiType=Rectangles  roiPortion=Entire ROI  roiOutput=Individual statistics for each ROI  roiFlag=off  roundingMode=Floor  overflowMode=off  outputDataTypeStr=Inherit: Same as accumulator  outputMin=[]  outputMax=[]  outputLastDataTypeStr=Inherit: Same as accumulator
  Mean5 : dspstat3/Mean  run=off  reset_popup=None  directionMode=Entire input  dimension=3  roiEnable=off  roiType=Rectangles  roiPortion=Entire ROI  roiOutput=Individual statistics for each ROI  roiFlag=off  roundingMode=Floor  overflowMode=off  outputDataTypeStr=Inherit: Same as accumulator  outputMin=[]  outputMax=[]  outputLastDataTypeStr=Inherit: Same as accumulator
  Mean6 : dspstat3/Mean  run=off  reset_popup=None  directionMode=Entire input  dimension=3  roiEnable=off  roiType=Rectangles  roiPortion=Entire ROI  roiOutput=Individual statistics for each ROI  roiFlag=off  roundingMode=Floor  overflowMode=off  outputDataTypeStr=Inherit: Same as accumulator  outputMin=[]  outputMax=[]  outputLastDataTypeStr=Inherit: Same as accumulator
  Scope : Scope  NumInputPorts=2
  Vector Concatenate : Concatenate  NumInputs=3
  mean_data : Outport
  wires:
  data/1 -> Demux/1, Scope/1
  Vector Concatenate/1 -> mean_data/1, Scope/2
  Mean4/1 -> Vector Concatenate/1
  Demux/3 -> Buffer2/1
  Buffer1/1 -> Mean5/1  "fby_buff"
  Demux/1 -> Buffer/1
  Buffer2/1 -> Mean6/1  "fbz_buff"
  Mean5/1 -> Vector Concatenate/2
  Buffer/1 -> Mean4/1  "fbx_buff"
  Demux/2 -> Buffer1/1
  Mean6/1 -> Vector Concatenate/3

== system main_RI_LIEKF_GNSSOutrage/State estimation/15dim KF1/INS propogation/Init_PVQ2/Subsystem1 ==
  data : Inport
  Buffer : Buffer  N=50  V=49  OutputFrames=off
  Buffer1 : Buffer  N=50  V=49  OutputFrames=off
  Buffer2 : Buffer  N=50  V=49  OutputFrames=off
  Demux : Demux  Outputs=3
  Mean4 : dspstat3/Mean  run=off  reset_popup=None  directionMode=Entire input  dimension=3  roiEnable=off  roiType=Rectangles  roiPortion=Entire ROI  roiOutput=Individual statistics for each ROI  roiFlag=off  roundingMode=Floor  overflowMode=off  outputDataTypeStr=Inherit: Same as accumulator  outputMin=[]  outputMax=[]  outputLastDataTypeStr=Inherit: Same as accumulator
  Mean5 : dspstat3/Mean  run=off  reset_popup=None  directionMode=Entire input  dimension=3  roiEnable=off  roiType=Rectangles  roiPortion=Entire ROI  roiOutput=Individual statistics for each ROI  roiFlag=off  roundingMode=Floor  overflowMode=off  outputDataTypeStr=Inherit: Same as accumulator  outputMin=[]  outputMax=[]  outputLastDataTypeStr=Inherit: Same as accumulator
  Mean6 : dspstat3/Mean  run=off  reset_popup=None  directionMode=Entire input  dimension=3  roiEnable=off  roiType=Rectangles  roiPortion=Entire ROI  roiOutput=Individual statistics for each ROI  roiFlag=off  roundingMode=Floor  overflowMode=off  outputDataTypeStr=Inherit: Same as accumulator  outputMin=[]  outputMax=[]  outputLastDataTypeStr=Inherit: Same as accumulator
  Vector Concatenate : Concatenate  NumInputs=3
  mean_data : Outport
  wires:
  Mean6/1 -> Vector Concatenate/3
  Demux/2 -> Buffer1/1
  Buffer/1 -> Mean4/1  "fbx_buff"
  Mean5/1 -> Vector Concatenate/2
  Buffer2/1 -> Mean6/1  "fbz_buff"
  Demux/1 -> Buffer/1
  Buffer1/1 -> Mean5/1  "fby_buff"
  Demux/3 -> Buffer2/1
  Mean4/1 -> Vector Concatenate/1
  Vector Concatenate/1 -> mean_data/1
  data/1 -> Demux/1

== system main_RI_LIEKF_GNSSOutrage/State estimation/15dim KF1/INS propogation/accl bias compensation/error compensation1 ==
  dda : Inport
  Add3 : Sum
  Memory1 : Memory
  da : Outport
  wires:
  dda/1 -> Add3/1
  Add3/1 -> da/1, Memory1/1
  Memory1/1 -> Add3/2

== system main_RI_LIEKF_GNSSOutrage/State estimation/15dim KF1/INS propogation/gyro bias compensation/error compensation ==
  ddg : Inport
  Enable : Inport  Port=2
  Add3 : Sum
  If Action Subsystem1 : Subsystem  TreatAsAtomicUnit=on
  If1 : If  IfExpression=u1 == 1  ShowElse=off
  Memory1 : Memory
  dg : Outport
  wires:
  ddg/1 -> Add3/1
  Enable/1 -> If1/1
  If1/1 -> If Action Subsystem1/Action
  Memory1/1 -> Add3/2
  Add3/1 -> dg/1, Memory1/1

== system main_RI_LIEKF_GNSSOutrage/State estimation/15dim KF1/INS propogation/vel_pos_update/Kinematic Equation ==
  Cbn : Inport
  Ab : Inport  Port=2
  Add : Sum  Inputs=+-
  Constant : Constant  Value=[0 0 -g0]  OutDataTypeStr=single
  Product : Product  Multiplication=Matrix(*)  RndMeth=Zero
  Scope : Scope
  Scope1 : Scope  NumInputPorts=2
  An : Outport
  wires:
  Cbn/1 -> Product/1
  Add/1 -> An/1, Scope1/2
  Ab/1 -> Product/2, Scope1/1
  Product/1 -> Scope/1, Add/1
  Constant/1 -> Add/2

== system main_RI_LIEKF_GNSSOutrage/State estimation/15dim KF1/INS propogation/vel_pos_update/pos update ==
  vel_k : Inport
  dp : Inport  Port=2
  QGC_init : Inport  Port=3
  p0 : Inport  Port=4
  Add1 : Sum  Inputs=++-
  Delay1 : Delay  DelayLength=1  InitialConditionSource=Input port  ExternalReset=Rising
      settings: InputPortMap=u0,r5,p4
  Gain1 : Gain  Gain=dt
  Reshape1 : Reshape  OutputDimensionality=Column vector (2-D)
  p_k : Outport
  wires:
  p0/1 -> Reshape1/1
  dp/1 -> Add1/3
  QGC_init/1 -> Delay1/2
  Add1/1 -> Delay1/1, p_k/1
  Reshape1/1 -> Delay1/3
  Delay1/1 -> Add1/2
  Gain1/1 -> Add1/1
  vel_k/1 -> Gain1/1

== system main_RI_LIEKF_GNSSOutrage/State estimation/15dim KF1/INS propogation/vel_pos_update/vel update ==
  QGC_init : Inport
  An : Inport  Port=2
  KFState_dv : Inport  Port=3
  v0 : Inport  Port=4
  Add : Sum  Inputs=++-
  Delay : Delay  DelayLength=1  InitialConditionSource=Input port  ExternalReset=Rising
      settings: InputPortMap=u0,r5,p4
  Gain : Gain  Gain=dt
  Reshape : Reshape  OutputDimensionality=Column vector (2-D)
  vel_k : Outport
  wires:
  QGC_init/1 -> Delay/2
  Reshape/1 -> Delay/3
  KFState_dv/1 -> Add/3
  An/1 -> Gain/1
  v0/1 -> Reshape/1
  Add/1 -> Delay/1, vel_k/1
  Gain/1 -> Add/1
  Delay/1 -> Add/2

== system main_RI_LIEKF_GNSSOutrage/State estimation/ER EKF/Error State Kalman Filter/Extended Kalman Filter1/Correct1 ==
  yMeas : Inport  SampleTime=SampleTime
  R : Inport  Port=2  SampleTime=SampleTime
  uMeas : Inport  Port=3  SampleTime=SampleTime
  uBlockOrdering : Inport  Port=4  SampleTime=SampleTime
  Enable : EnablePort
  Correct : MATLAB Function  TreatAsAtomicUnit=on
  Data Store ReadP : DataStoreRead  DataStoreName=P  IndexOptions=Index vector (dialog)  Indices=1  OutputSizes=1
  Data Store ReadX : DataStoreRead  DataStoreName=x  IndexOptions=Index vector (dialog)  Indices=1  OutputSizes=1
  Data Store WriteP : DataStoreWrite  DataStoreName=P  IndexOptions=Index vector (dialog)  Indices=1  OutputSizes=1
  Data Store WriteX : DataStoreWrite  DataStoreName=x  IndexOptions=Index vector (dialog)  Indices=1  OutputSizes=1
  RegisterSimulinkFcn : S-Function  FunctionName=ekfukfRegisterSimulinkFcn  Parameters=int32(3), 1, pM.HasAdditiveNoise, SampleTime, DataType, SLFcnsToRegister  SFunctionDeploymentMode=off  EnableBusSupport=off
  yBlockOrdering : Outport  VectorParamsAs1DForOutWhenUnconnected=off
  wires:
  Data Store ReadX/1 -> RegisterSimulinkFcn/1, Correct/1(x)
  Data Store ReadP/1 -> Correct/2("P ")
  Correct/2(P) -> Data Store WriteP/1
  R/1 -> Correct/4(R), RegisterSimulinkFcn/3
  Correct/1(xNew) -> Data Store WriteX/1
  Correct/3(blockOrdering) -> yBlockOrdering/1
  uBlockOrdering/1 -> Correct/6("blockOrdering ")
  uMeas/1 -> Correct/5(uMeas)
  yMeas/1 -> RegisterSimulinkFcn/2, Correct/3(yMeas)

== system main_RI_LIEKF_GNSSOutrage/State estimation/ER EKF/Error State Kalman Filter/Extended Kalman Filter1/Output ==
  uBlockOrdering : Inport
  Data Store Read : DataStoreRead  DataStoreName=x  IndexOptions=Index vector (dialog)  Indices=1  OutputSizes=1
  Data Store Read1 : DataStoreRead  DataStoreName=P  IndexOptions=Index vector (dialog)  Indices=1  OutputSizes=1
  MATLAB Function : MATLAB Function  TreatAsAtomicUnit=on
  x : Outport  VectorParamsAs1DForOutWhenUnconnected=off
  P : Outport  Port=2  VectorParamsAs1DForOutWhenUnconnected=off
  yBlockOrdering : Outport  Port=3  VectorParamsAs1DForOutWhenUnconnected=off
  wires:
  Data Store Read/1 -> x/1
  Data Store Read1/1 -> MATLAB Function/1(S)
  uBlockOrdering/1 -> yBlockOrdering/1
  MATLAB Function/1(P) -> P/1

== system main_RI_LIEKF_GNSSOutrage/State estimation/ER EKF/Error State Kalman Filter/Extended Kalman Filter1/Predict ==
  Q : Inport  SampleTime=SampleTime
  uState : Inport  Port=2  SampleTime=SampleTime
  uBlockOrdering : Inport  Port=3  SampleTime=SampleTime
  Data Store Read1 : DataStoreRead  Commented=on  DataStoreName=feedback_flag_18dim  IndexOptions=Index vector (dialog)  Indices=1  OutputSizes=1
  Data Store Write : DataStoreWrite  DataStoreName=P  IndexOptions=Index vector (dialog)  Indices=1  OutputSizes=1
  Data Store Write1 : DataStoreWrite  DataStoreName=x  IndexOptions=Index vector (dialog)  Indices=1  OutputSizes=1
  Data Store WriteX : DataStoreWrite  DataStoreName=x  IndexOptions=Index vector (dialog)  Indices=1  OutputSizes=1
  Data Store ReadP : DataStoreRead  DataStoreName=P  IndexOptions=Index vector (dialog)  Indices=1  OutputSizes=1
  Data Store ReadX : DataStoreRead  DataStoreName=x  IndexOptions=Index vector (dialog)  Indices=1  OutputSizes=1
  If : If  Commented=on  IfExpression=u1 == 1  ShowElse=off
  If Action Subsystem : Subsystem  Commented=on  TreatAsAtomicUnit=on
  Predict : MATLAB Function  TreatAsAtomicUnit=on
  RegisterSimulinkFcn : S-Function  FunctionName=ekfukfRegisterSimulinkFcn  Parameters=int32(2), 0, pS.HasAdditiveNoise, SampleTime, DataType, SLFcnsToRegister  SFunctionDeploymentMode=off  EnableBusSupport=off
  Zero : Constant  Value=zeros(15,1)  OutDataTypeStr=Inherit: Inherit via back propagation
  wires:
  Data Store ReadP/1 -> Predict/2("P ")
  Predict/2(P) -> Data Store Write/1
  Q/1 -> Predict/3(Q), RegisterSimulinkFcn/2
  Predict/1(xNew) -> Data Store WriteX/1
  Data Store ReadX/1 -> Predict/1(x), RegisterSimulinkFcn/1
  uBlockOrdering/1 -> Predict/5(unused)
  uState/1 -> Predict/4(uState)
  Data Store Read1/1 -> If/1
  If/1 -> If Action Subsystem/Action
  Zero/1 -> Data Store Write1/1

== system main_RI_LIEKF_GNSSOutrage/State estimation/ER EKF/Error State Kalman Filter/Simulink Function - State Transition/Cal Phi ==
  <DCM_b_n> : Inport
  wxyz : Inport  Port=2
  axyz : Inport  Port=3
  Constant : Constant  Value=dt
  MATLAB Function1 : MATLAB Function  TreatAsAtomicUnit=on
  Transpose : Math  Operator=transpose
  Phi : Outport
  wires:
  <DCM_b_n>/1 -> Transpose/1
  MATLAB Function1/1(Phi) -> Phi/1
  wxyz/1 -> MATLAB Function1/3(wxyz)
  axyz/1 -> MATLAB Function1/1(axyz)
  Constant/1 -> MATLAB Function1/4(dt)
  Transpose/1 -> MATLAB Function1/2(Cnb)

== system main_RI_LIEKF_GNSSOutrage/State estimation/ER EKF/Error State Kalman Filter/Simulink Function - State Transition Jacobian/Cal Phi1 ==
  <DCM_b_n> : Inport
  wxyz : Inport  Port=2
  axyz : Inport  Port=3
  Constant : Constant  Value=dt
  MATLAB Function1 : MATLAB Function  TreatAsAtomicUnit=on
  Transpose : Math  Operator=transpose
  Phi : Outport
  wires:
  <DCM_b_n>/1 -> Transpose/1
  MATLAB Function1/1(Phi) -> Phi/1
  wxyz/1 -> MATLAB Function1/3(wxyz)
  axyz/1 -> MATLAB Function1/1(axyz)
  Constant/1 -> MATLAB Function1/4(dt)
  Transpose/1 -> MATLAB Function1/2(Cnb)
